simulink model "System_Design_OQPSK"  (R2023b)
settings: Solver=FixedStepDiscrete  StartTime=0.0  StopTime=(16+4+1)*24-1  RelTol=1e-3
libraries: dspsigops x2, commchan3 x1, dspsrcs4 x1
settings Model: LastModifiedBy=AMEY THAKUR

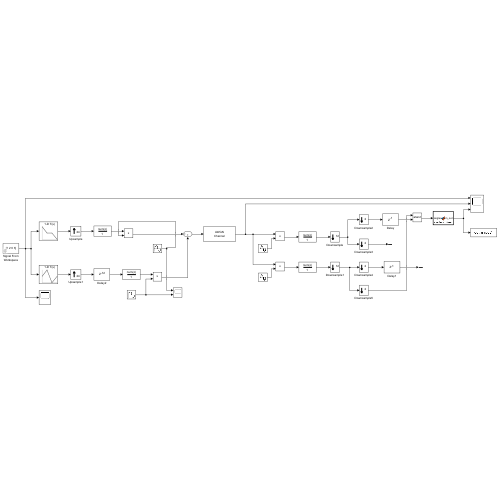
[thumbnail: Simulink's stored preview of the top-level diagram]
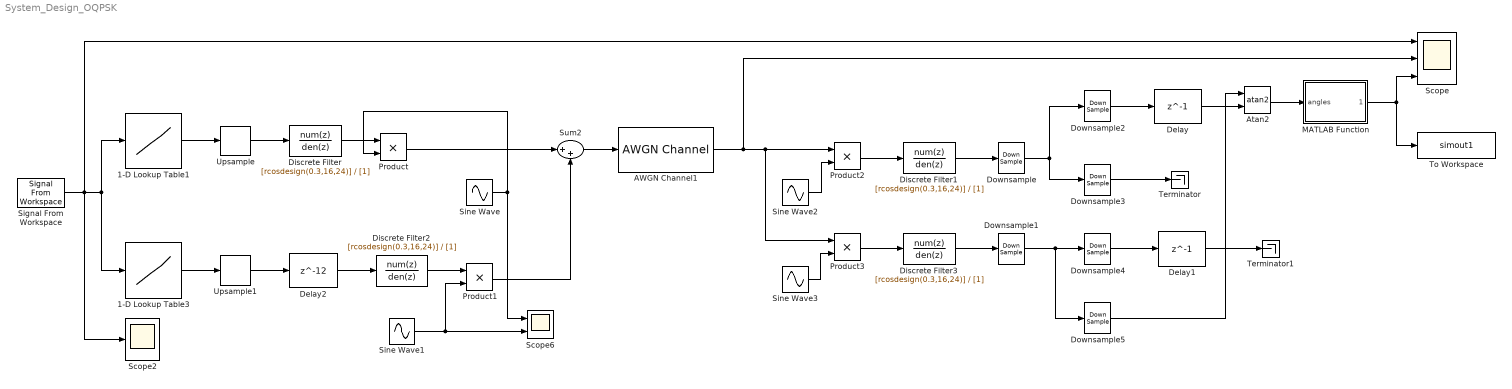
== system System_Design_OQPSK ==
  1-D Lookup Table1 : Lookup_n-D  NumberOfTableDimensions=1  BreakpointsForDimension1=[0 1 2 3]  Table=[3 0 0 -3]  InternalRulePriority=Speed  RndMeth=Simplest
  1-D Lookup Table3 : Lookup_n-D  NumberOfTableDimensions=1  BreakpointsForDimension1=[0 1 2 3]  Table=[0 3 -3 0]  InternalRulePriority=Speed  RndMeth=Simplest
  AWGN Channel1 : commchan3/AWGN Channel  LegacyMode=on  NoiseMethod="Signal to noise ratio  (SNR)"  noiseMode="Signal to noise ratio  (Eb/No)"  EbNo=40  EsNo=10  SNR=10  BitsPerSymbol=1  SignalPower=1  SamplesPerSymbol=1  SymbolPeriod=1  VarianceSource=Parameter  Variance=1  RandomStream=Global stream  Seed=110107589  SimulateUsing=Code generation
  Atan2 : Trigonometry  Operator=atan2
  Delay : Delay  DelayLength=1  InitialCondition=0  UseCircularBuffer=on  SampleTime=1
  Delay1 : Delay  DelayLength=1  InitialCondition=0  UseCircularBuffer=on  SampleTime=1
  Delay2 : Delay  DelayLength=12  InitialCondition=0  UseCircularBuffer=on  SampleTime=1
  Discrete Filter{,1..3} (4 alike) : DiscreteFilter  Numerator=[rcosdesign(0.3,16,24)]  Denominator=[1]
  Downsample : DownSample  N=12  RateOptions=Allow multirate processing
  Downsample1 : DownSample  N=12  RateOptions=Allow multirate processing
  Downsample2 : DownSample  RateOptions=Allow multirate processing
  Downsample3 : DownSample  phase=1  RateOptions=Allow multirate processing
  Downsample4 : DownSample  RateOptions=Allow multirate processing
  Downsample5 : DownSample  phase=1  RateOptions=Allow multirate processing
  MATLAB Function : MATLAB Function  TreatAsAtomicUnit=on
  Product{,1..3} (4 alike) : Product
  Scope : Scope  NumInputPorts=3
  Scope2 : Scope
  Scope6 : Scope  NumInputPorts=2
  Signal From Workspace : dspsrcs4/Signal From Workspace  X=[1 2 0 3]  Ts=24  nsamps=1  OutputAfterFinalValue=Setting to zero  ignoreOrWarnInputAndFrameLengths=off  OutputFrames=off
  Sine Wave : Sin  Amplitude=sqrt(2)  Frequency=2*pi*0.25  Phase=pi/2  SampleTime=1
  Sine Wave1 : Sin  Amplitude=-sqrt(2)  Frequency=2*pi*0.25  SampleTime=1
  Sine Wave2 : Sin  Amplitude=sqrt(2)  Frequency=2*pi*0.25  Phase=pi/2  SampleTime=1
  Sine Wave3 : Sin  Amplitude=-sqrt(2)  Frequency=2*pi*0.25  SampleTime=1
  Sum2 : Sum  Inputs=|++
  Terminator : Terminator
  Terminator1 : Terminator
  To Workspace : ToWorkspace  VariableName=simout1  SaveFormat=Timeseries  SampleTime=-1
  Upsample : dspsigops/Upsample  FactorSource=Dialog parameter  N=24  Nmax=16  phase=0  RateOptions=Allow multirate processing  ic=0  mode=Unused parameter value
  Upsample1 : dspsigops/Upsample  FactorSource=Dialog parameter  N=24  Nmax=16  phase=0  RateOptions=Allow multirate processing  ic=0  mode=Unused parameter value
  wires:
  1-D Lookup Table1/1 -> Upsample/1
  Upsample/1 -> Discrete Filter/1
  Signal From Workspace/1 -> Scope2/1, Scope/1, 1-D Lookup Table1/1, 1-D Lookup Table3/1
  Product/1 -> Sum2/1
  Product1/1 -> Sum2/2
  Sine Wave1/1 -> Product1/2, Scope6/2
  1-D Lookup Table3/1 -> Upsample1/1
  Sine Wave/1 -> Product/2, Scope6/1
  Discrete Filter/1 -> Product/1
  Sum2/1 -> AWGN Channel1/1
  Discrete Filter2/1 -> Product1/1
  Downsample2/1 -> Delay/1
  MATLAB Function/1(sym_out) -> To Workspace/1, Scope/3
  Atan2/1 -> MATLAB Function/1(angles)
  Sine Wave2/1 -> Product2/2
  Sine Wave3/1 -> Product3/2
  Product3/1 -> Discrete Filter3/1
  Discrete Filter3/1 -> Downsample1/1
  Downsample4/1 -> Delay1/1
  Discrete Filter1/1 -> Downsample/1
  Product2/1 -> Discrete Filter1/1
  Downsample1/1 -> Downsample5/1, Downsample4/1
  Downsample3/1 -> Terminator/1
  Downsample/1 -> Downsample3/1, Downsample2/1
  Delay/1 -> Atan2/2
  AWGN Channel1/1 -> Scope/2, Product3/1, Product2/1
  Upsample1/1 -> Delay2/1
  Delay2/1 -> Discrete Filter2/1
  Delay1/1 -> Terminator1/1
  Downsample5/1 -> Atan2/1

== matlab function System_Design_OQPSK/MATLAB Function ==
  data: angles input; sym_out output
function sym_out = extract_symbols_from_angles(angles)

sym_out = zeros(size(angles));

for k = 1:length(angles)
    if angles(k) >= -pi/4 && angles(k) <= pi/4
        sym_out(k) = 0;
    elseif angles(k) >= pi/4 && angles(k) <= 3*pi/4
        sym_out(k) = 1;
    elseif angles(k) >= -3*pi/4 && angles(k) <= -pi/4
        sym_out(k) = 2;
    else
        sym_out(k) = 3;
    end
end
end
